simulink model "GPS_Tests"  (R2024a)
settings: Solver=VariableStepAuto  StartTime=0.0  StopTime=2  RelTol=1e-3
libraries: sensorgpslib x1
settings Model: Creator=gerar  LastModifiedBy=gerar

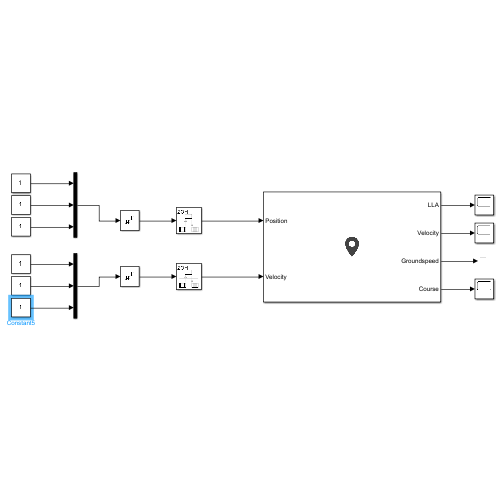
[thumbnail: Simulink's stored preview of the top-level diagram]
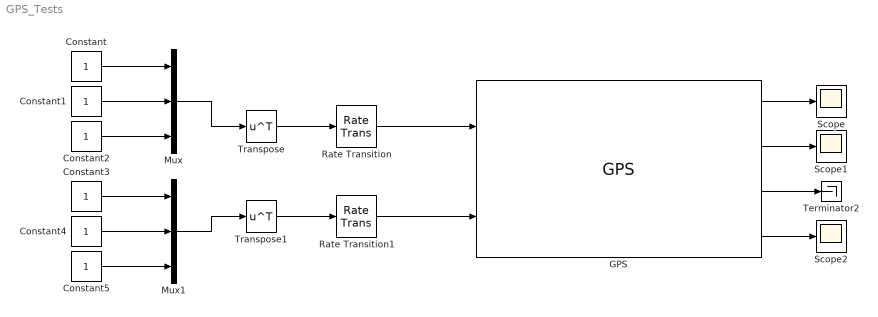
== system GPS_Tests ==
  Constant{,1..5} (6 alike) : Constant
  GPS : sensorgpslib/GPS  DispRefFrame=ENU  PositionInputFormat=Local  ReferenceLocation=[ 0, 0, 0 ]  HorizontalPositionAccuracy=1.6  VerticalPositionAccuracy=3  VelocityAccuracy=0.1  DecayFactor=0.999  SeedDouble=67  SimulateUsing=Interpreted execution
      settings: LibrarySourceBlock=mspsensorlib/GPS
  Mux : Mux  Inputs=3
  Mux1 : Mux  Inputs=3
  Rate Transition : RateTransition  OutPortSampleTime=0.01
  Rate Transition1 : RateTransition  OutPortSampleTime=0.01
  Scope : Scope
  Scope1 : Scope
  Scope2 : Scope
  Terminator2 : Terminator
  Transpose : Math  Operator=transpose
  Transpose1 : Math  Operator=transpose
  wires:
  GPS/3 -> Terminator2/1
  GPS/1 -> Scope/1
  GPS/2 -> Scope1/1
  GPS/4 -> Scope2/1
  Transpose1/1 -> Rate Transition1/1
  Transpose/1 -> Rate Transition/1
  Constant1/1 -> Mux/2
  Constant2/1 -> Mux/3
  Mux/1 -> Transpose/1
  Mux1/1 -> Transpose1/1
  Constant5/1 -> Mux1/3
  Constant3/1 -> Mux1/1
  Constant/1 -> Mux/1
  Constant4/1 -> Mux1/2
  Rate Transition/1 -> GPS/1
  Rate Transition1/1 -> GPS/2
